simulink model "robot_pose"  (R2022a)
settings: Solver=VariableStepAuto  StartTime=0.0  StopTime=Inf  RelTol=1e-3
libraries: robotlib x1
settings Model: Creator=sokajima  LastModifiedBy=sokajima

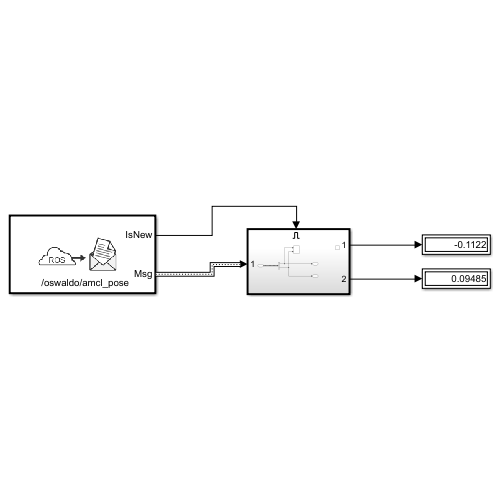
[thumbnail: Simulink's stored preview of the top-level diagram]
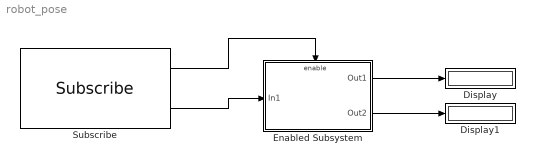
== system robot_pose ==
  Display : Display
  Display1 : Display
  Enabled Subsystem : Subsystem
  Subscribe : robotlib/Subscribe  topicSource=Specify your own  topic=/oswaldo/amcl_pose  messageType=geometry_msgs/PoseWithCovarianceStamped  SampleTime=0.03  legacyBusStruct=off  messageQueueLength=1
  wires:
  Subscribe/2 -> Enabled Subsystem/1(In1)
  Subscribe/1 -> Enabled Subsystem/Enable
  Enabled Subsystem/2(Out2) -> Display1/1
  Enabled Subsystem/1(Out1) -> Display/1

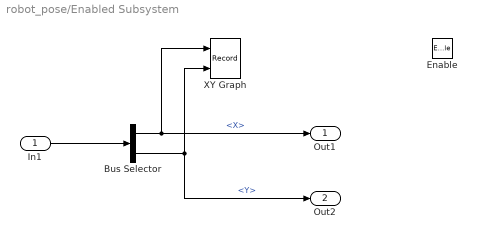
== system robot_pose/Enabled Subsystem ==
  In1 : Inport
  Enable : EnablePort
  Bus Selector : BusSelector  DialogController=Simulink.DDGSource_BusSelector  OutputSignals=Pose.Pose.Position.X,Pose.Pose.Position.Y
  XY Graph : Record  FileSettingsInternal="{\"entries\":[{\"content\":{\"excelSettings\":{\"content\":{},\"type\":\"Streamout.ExcelSettings\"}},\"type\":\"Streamout.FileSettingStorage\",\"uuid\":\"f322e8a0-ae82-4ecf-8768-dabf346e6e6b\"}],\"packageUris\":[\"http://schema.mathworks.com/mf0/streamout_blocks/R2020a\"],\"version\":\"1.0\"}"  Layout=[1 1]  SignalsInternal="{\"entries\":[{\"content\":{\"signals\":[{\"content\":{\"blockPath\":[\"robot_pose/Enabled Subsystem/XY Graph\"],\"channel\":[],\"dimensions\":[1],\"domain\":\"robot_pose/Enabled Subsystem/XY Graph\",\"lineColor\":\"#a2142f\",\"plots\":[1],\"port\":1,\"sid\":[\"\"],\"signalID\":218,\"signalName\":\"<X>\"},\"type\":\"RecordBlkView.Signal\",\"uuid\":\"7e22e004-de9a-4aba-88bd-710681b13f9e\"},{\"content\":{\"blockPath\":[\"robot_pose/Enabled Subsystem/XY Graph\"],\"channel\":[],\"dimensions\":[1],\"domain\":\"robot_pose/Enabled Subsystem/XY Graph\",\"lineColor\":\"#139fff\",\"plots\":[1],\"port\":2,\"sid\":[\"\"],\"signalID\":222,\"signalName\":\"<Y>\"},\"type\":\"RecordBlkView.Signal\",\"uuid\":\"c3d303d5-d31e-4095-b537-cb066a1a505d\"}]},\"type\":\"RecordBlkView.InputSignals\",\"uuid\":\"9259184b-0c6f-4629-ad28-23cd3b22c4c6\"}],\"packageUris\":[\"http://schema.mathworks.com/mf0/streamout_blocks/R2020a\"],\"version\":\"1.0\"}"  VisualizationBindings="{\"xyplotplugin\":{\"info\":[{\"series\":[{\"bindingParametersList\":[{\"parameter\":\"X-Axis\",\"signalID\":218,\"signalName\":\"<X>\"},{\"parameter\":\"Y-Axis\",\"signalID\":222,\"signalName\":\"<Y>\"}],\"seriesID\":23985}],\"subplotID\":1}]}}"  CompatibilityTag=XY  st=-1
  Out1 : Outport  VectorParamsAs1DForOutWhenUnconnected=off
  Out2 : Outport  Port=2  VectorParamsAs1DForOutWhenUnconnected=off
  wires:
  In1/1 -> Bus Selector/1
  Bus Selector/2 -> Out2/1, XY Graph/2  "<Y>"
  Bus Selector/1 -> Out1/1, XY Graph/1  "<X>"
